simulink model "GPESTN1_GPEDBS"  (Simulink 6.1)
settings: Solver=ode45  StartTime=0.0  StopTime=1000.0  MaxStep=0.01  MinStep=0.005  RelTol=1e-3
values from neighbouring files (symbols this model uses):
  A_gpe = 2    [data_GPE.m]    (also in data_GPI.m)
  A_stn = 5    [data_GPI.m]    (also in data_STN.m)
  B_gpe = .08    (= 0.08)    [data_GPE.m]    (also in data_GPI.m)
  B_stn = 1    [data_GPI.m]    (also in data_STN.m)
  c_gpe = 1    [data_GPE.m]
  c_stn = 1    [data_STN.m]
  cag0 = i_v_16(177:192)    [launch_sysGPESTN1.m]    (also in launch_sysGPESTN1_GPEDBS.m)
  cas0 = i_v_16(65:80)    [launch_sysGPESTN1.m]    (also in launch_sysGPESTN1_GPEDBS.m)
  egpegpe = -80    [data_synapses.m]
  egpestn = -100    [data_synapses.m]
  ek_gpe = -80.0    (= -80)    [data_GPE.m]
  ek_stn = -80.0    (= -80)    [data_STN.m]
  el_gpe = -55.0    (= -55)    [data_GPE.m]
  el_stn = -60.0    (= -60)    [data_STN.m]
  epsil_gpe = 1*10^-4    (= 0.0001)    [data_GPE.m]
  epsil_stn = 3.75*10^-5    (= 3.75e-05)    [data_STN.m]
  estngpe = 0    [data_synapses.m]
  gahp_gpe = 30.0    (= 30)    [data_GPE.m]
  gahp_stn = 9.0    (= 9)    [data_STN.m]
  gca_gpe = 0.1    [data_GPE.m]
  gca_stn = 0.5    [data_STN.m]
  ggpegpe = .3    (= 0.3)    [data_synapses.m]    (also in launch_sysGPESTN1.m; launch_sysGPESTN1_GPEDBS.m = 0)
  ggpestn = .90    (= 0.9)    [data_synapses.m]
  gk_gpe = 30.0    (= 30)    [data_GPE.m]
  gk_stn = 45.0    (= 45)    [data_STN.m]
  gl_gpe = .1    (= 0.1)    [data_GPE.m]
  gl_stn = 2.25    [data_STN.m]
  gna_gpe = 120    [data_GPE.m]
  gna_stn = 37.5    [data_STN.m]
  gstngpe = .3    (= 0.3)    [data_synapses.m]
  gt_gpe = .5    (= 0.5)    [data_GPE.m]
  gt_stn = 0.5    [data_STN.m]
  hg0 = i_v_16(129:144)    [launch_sysGPESTN1.m]    (also in launch_sysGPESTN1_GPEDBS.m)
  hs0 = i_v_16(17:32)    [launch_sysGPESTN1.m]    (also in launch_sysGPESTN1_GPEDBS.m)
  k1_gpe = 30.0    (= 30)    [data_GPE.m]
  k1_stn = 15.0    (= 15)    [data_STN.m]
  kca_gpe = 15    [data_GPE.m]
  kca_stn = 22.5    [data_STN.m]
  ng0 = i_v_16(145:160)    [launch_sysGPESTN1.m]    (also in launch_sysGPESTN1_GPEDBS.m)
  ns0 = i_v_16(33:48)    [launch_sysGPESTN1.m]    (also in launch_sysGPESTN1_GPEDBS.m)
  phih_gpe = 0.05    [data_GPE.m]
  phih_stn = 0.75    [data_STN.m]
  phin_gpe = 0.1    [data_GPE.m]
  phin_stn = 0.75    [data_STN.m]
  phir_gpe = 1    [data_GPE.m]
  phir_stn = 0.5    [data_STN.m]
  rg0 = i_v_16(161:176)    [launch_sysGPESTN1.m]    (also in launch_sysGPESTN1_GPEDBS.m)
  rs0 = i_v_16(49:64)    [launch_sysGPESTN1.m]    (also in launch_sysGPESTN1_GPEDBS.m)
  sg0 = i_v_16(193:208)    [launch_sysGPESTN1.m]    (also in launch_sysGPESTN1_GPEDBS.m)
  sigmaa_gpe = 2    [data_GPE.m]
  sigmaa_stn = 7.8    [data_STN.m]
  sigmab_stn = -0.07    [data_STN.m]
  sigmagh_gpe = 2.0    (= 2)    [data_GPE.m]
  sigmagh_stn = 8.0    (= 8)    [data_STN.m]
  sigmah_gpe = -12    [data_GPE.m]
  sigmah_stn = -3.1    [data_STN.m]
  sigmam_gpe = 10.0    (= 10)    [data_GPE.m]
  sigmam_stn = 15.0    (= 15)    [data_STN.m]
  sigman_gpe = 14.0    (= 14)    [data_GPE.m]
  sigman_stn = 8.0    (= 8)    [data_STN.m]
  sigmar_gpe = -2.0    (= -2)    [data_GPE.m]
  sigmar_stn = -2.0    (= -2)    [data_STN.m]
  sigmas_gpe = 2    [data_GPE.m]
  sigmas_stn = 8.0    (= 8)    [data_STN.m]
  sigmatauh_gpe = -12    [data_GPE.m]
  sigmatauh_stn = -3.0    (= -3)    [data_STN.m]
  sigmataun_gpe = -12.0    (= -12)    [data_GPE.m]
  sigmataun_stn = -26.0    (= -26)    [data_STN.m]
  sigmataur_stn = -2.2    [data_STN.m]
  ss0 = i_v_16(81:96)    [launch_sysGPESTN1.m]    (also in launch_sysGPESTN1_GPEDBS.m)
  syn_stngpe_gain = .2    (= 0.2)    [data_STN.m]
  tauh0_gpe = .05    (= 0.05)    [data_GPE.m]
  tauh0_stn = 1.0    (= 1)    [data_STN.m]
  tauh1_gpe = .27    (= 0.27)    [data_GPE.m]
  tauh1_stn = 500.0    (= 500)    [data_STN.m]
  taun0_gpe = .05    (= 0.05)    [data_GPE.m]
  taun0_stn = 1.0    (= 1)    [data_STN.m]
  taun1_gpe = .27    (= 0.27)    [data_GPE.m]
  taun1_stn = 100.0    (= 100)    [data_STN.m]
  taur0_stn = 7.1    [data_STN.m]
  taur1_stn = 17.5    [data_STN.m]
  taur_gpe = 30.0    (= 30)    [data_GPE.m]
  theta_gpe = 20    [data_GPE.m]    (also in data_GPI.m)
  theta_stn = 30    [data_GPI.m]    (also in data_STN.m)
  thetaa_gpe = -57.0    (= -57)    [data_GPE.m]
  thetaa_stn = -63.0    (= -63)    [data_STN.m]
  thetab_stn = 0.25    [data_STN.m]
  thetagh_gpe = -57.0    (= -57)    [data_GPE.m]
  thetagh_stn = -39.0    (= -39)    [data_STN.m]
  thetah_gpe = -58.0    (= -58)    [data_GPE.m]
  thetah_stn = -39.0    (= -39)    [data_STN.m]
  thetam_gpe = -37.0    (= -37)    [data_GPE.m]
  thetam_stn = -30.0    (= -30)    [data_STN.m]
  thetan_gpe = -50.0    (= -50)    [data_GPE.m]
  thetan_stn = -32.0    (= -32)    [data_STN.m]
  thetar_gpe = -70.0    (= -70)    [data_GPE.m]
  thetar_stn = -67.0    (= -67)    [data_STN.m]
  thetas_gpe = -35.0    (= -35)    [data_GPE.m]
  thetas_stn = -39.0    (= -39)    [data_STN.m]
  thetatauh_gpe = -40.0    (= -40)    [data_GPE.m]
  thetatauh_stn = -57.0    (= -57)    [data_STN.m]
  thetataun_gpe = -40.0    (= -40)    [data_GPE.m]
  thetataun_stn = -80.0    (= -80)    [data_STN.m]
  thetataur_stn = 68.0    (= 68)    [data_STN.m]
  vg0 = i_v_16(113:128)    [launch_sysGPESTN1.m]    (also in launch_sysGPESTN1_GPEDBS.m)
  vs0 = i_v_16(1:16)    [launch_sysGPESTN1.m]    (also in launch_sysGPESTN1_GPEDBS.m)
undefined symbols (not defined in the file or in its folder): cag01, cas01, hg01, hs01, ng01, ns01, rg01, rs01, sg01, ss01, vg01, vs01
(part 1 of 9)
settings Model: LastModifiedBy=marco  ExtModeAutoUpdateStatusClock=off
settings DataIOCC: SignalLoggingName=sigsOut
settings OptimizationCC: BooleanDataType=off  InlineInvariantSignals=off
settings HardwareCC: TargetUnknown=on

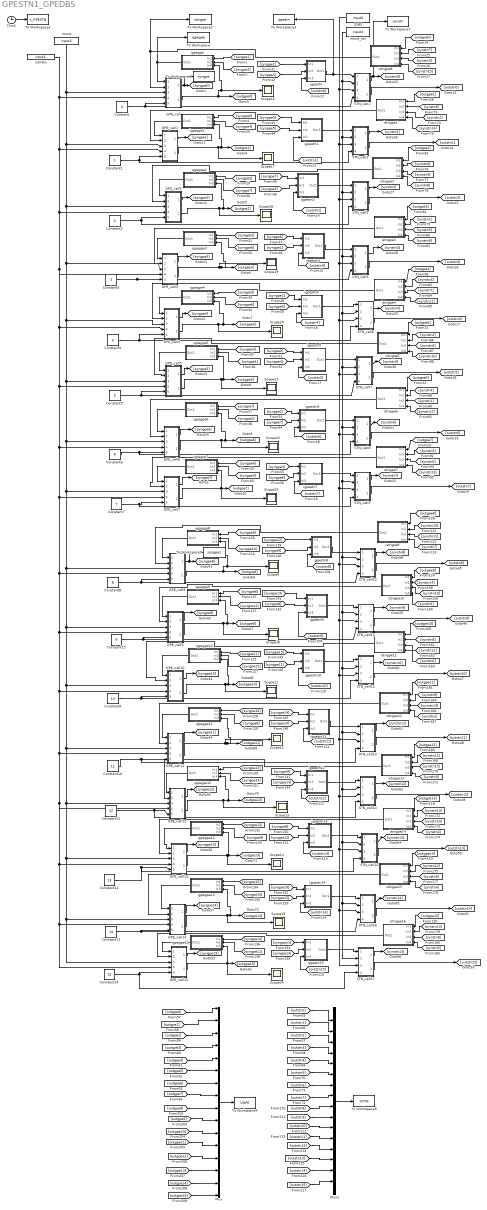
== system GPESTN1_GPEDBS ==
  Clock : Clock
      settings: Decimation=10
  Constant : Constant  Value=0
  Constant1 : Constant
  Constant10 : Constant  Value=11
  Constant11 : Constant  Value=12
  Constant12 : Constant  Value=13
  Constant13 : Constant  Value=14
  Constant14 : Constant  Value=15
  Constant15 : Constant  Value=9
  Constant2 : Constant  Value=2
  Constant3 : Constant  Value=3
  Constant4 : Constant  Value=4
  Constant5 : Constant  Value=5
  Constant6 : Constant  Value=6
  Constant7 : Constant  Value=7
  Constant8 : Constant  Value=8
  Constant9 : Constant  Value=10
  GPE_cell : Subsystem
  GPE_cell1 : Subsystem
  GPE_cell10 : Subsystem
  GPE_cell11 : Subsystem
  GPE_cell12 : Subsystem
  GPE_cell13 : Subsystem
  GPE_cell14 : Subsystem
  GPE_cell15 : Subsystem
  GPE_cell2 : Subsystem
  GPE_cell3 : Subsystem
  GPE_cell4 : Subsystem
  GPE_cell5 : Subsystem
  GPE_cell6 : Subsystem
  GPE_cell7 : Subsystem
  GPE_cell8 : Subsystem
  GPE_cell9 : Subsystem
  IDBS : FromWorkspace  Orientation=left  VariableName=input3  SampleTime=0.01
  Mux : Mux  Inputs=16
  Mux1 : Mux  Inputs=16
  STN_cell1 : Subsystem
  STN_cell10 : Subsystem
  STN_cell11 : Subsystem
  STN_cell12 : Subsystem
  STN_cell13 : Subsystem
  STN_cell14 : Subsystem
  STN_cell15 : Subsystem
  STN_cell16 : Subsystem
  STN_cell17 : Subsystem
  STN_cell2 : Subsystem
  STN_cell3 : Subsystem
  STN_cell5 : Subsystem
  STN_cell6 : Subsystem
  STN_cell7 : Subsystem
  STN_cell8 : Subsystem
  STN_cell9 : Subsystem
  Scope{9..24} (16 alike) : Scope
      Scope10 settings: YMin=-125  YMax=75  SaveName=ScopeData9
      Scope11 settings: YMin=-80  YMax=60  SaveName=ScopeData10
      Scope12 settings: YMin=-250  YMax=100  SaveName=ScopeData11
      Scope13 settings: YMin=-100  YMax=60  SaveName=ScopeData12
      Scope14 settings: YMin=-80  YMax=60  SaveName=ScopeData13
      Scope15 settings: YMin=-250  YMax=100  SaveName=ScopeData14
      Scope16 settings: YMin=-80  YMax=60
      Scope17 settings: YMin=-80  YMax=60  SaveName=ScopeData16
      Scope18 settings: YMin=-80  YMax=60  SaveName=ScopeData17
      Scope19 settings: YMin=-80  YMax=60  SaveName=ScopeData18
      Scope20 settings: SaveName=ScopeData19
      Scope21 settings: YMin=-80  YMax=60  SaveName=ScopeData20
      Scope22 settings: YMin=-80  YMax=60  SaveName=ScopeData21
      Scope23 settings: YMin=-80  YMax=60  SaveName=ScopeData22
      Scope24 settings: YMin=-80  YMax=60  SaveName=ScopeData15
      Scope9 settings: YMin=-90  YMax=60  SaveName=ScopeData23
  To Workspace : ToWorkspace  VariableName=igpegpe  SampleTime=-1  SaveFormat=Array
  To Workspace1 : ToWorkspace  VariableName=t_GPESTN  SampleTime=-1  SaveFormat=Array
  To Workspace2 : ToWorkspace  VariableName=istngpe  SampleTime=-1  SaveFormat=Array
  To Workspace3 : ToWorkspace  VariableName=igpestn  SampleTime=-1  SaveFormat=Array
  To Workspace4 : ToWorkspace  VariableName=VGPE  SampleTime=-1  SaveFormat=Array
  To Workspace5 : ToWorkspace  VariableName=VSTN  SampleTime=-1  SaveFormat=Array
  To Workspace6 : ToWorkspace  VariableName=syngpe  SampleTime=-1  SaveFormat=Array
  To Workspace7 : ToWorkspace  VariableName=synstn  SampleTime=-1  SaveFormat=Array
  To Workspace9 : ToWorkspace  VariableName=syngpe1  SampleTime=-1  SaveFormat=Array
  igpegpe : Subsystem  Orientation=left
  igpegpe1 : Subsystem  Orientation=left
  igpegpe10 : Subsystem  Orientation=left
  igpegpe11 : Subsystem  Orientation=left
  igpegpe12 : Subsystem  Orientation=left
  igpegpe13 : Subsystem  Orientation=left
  igpegpe14 : Subsystem  Orientation=left
  igpegpe15 : Subsystem  Orientation=left
  igpegpe2 : Subsystem  Orientation=left
  igpegpe3 : Subsystem  Orientation=left
  igpegpe4 : Subsystem  Orientation=left
  igpegpe5 : Subsystem  Orientation=left
  igpegpe6 : Subsystem  Orientation=left
  igpegpe7 : Subsystem  Orientation=left
  igpegpe8 : Subsystem  Orientation=left
  igpegpe9 : Subsystem  Orientation=left
  igpestn : Subsystem
  igpestn1 : Subsystem
  igpestn10 : Subsystem
  igpestn11 : Subsystem
  igpestn12 : Subsystem
  igpestn13 : Subsystem
  igpestn14 : Subsystem
  igpestn15 : Subsystem
  igpestn2 : Subsystem
  igpestn3 : Subsystem
  igpestn4 : Subsystem
  igpestn5 : Subsystem
  igpestn6 : Subsystem
  igpestn7 : Subsystem
  igpestn8 : Subsystem
  igpestn9 : Subsystem
  imore : FromWorkspace  Orientation=down  VariableName=input2  SampleTime=1
  imore_stn : FromWorkspace  Orientation=left  VariableName=input4  SampleTime=1
  istngpe1 : Subsystem  Orientation=left
  istngpe10 : Subsystem  Orientation=left
  istngpe11 : Subsystem  Orientation=left
  istngpe12 : Subsystem  Orientation=left
  istngpe13 : Subsystem  Orientation=left
  istngpe14 : Subsystem  Orientation=left
  istngpe15 : Subsystem  Orientation=left
  istngpe16 : Subsystem  Orientation=left
  istngpe2 : Subsystem  Orientation=left
  istngpe3 : Subsystem  Orientation=left
  istngpe4 : Subsystem  Orientation=left
  istngpe5 : Subsystem  Orientation=left
  istngpe6 : Subsystem  Orientation=left
  istngpe7 : Subsystem  Orientation=left
  istngpe8 : Subsystem  Orientation=left
  istngpe9 : Subsystem  Orientation=left
  istriato : FromWorkspace  VariableName=input1  SampleTime=1
  wires:
  Clock/1 -> To Workspace1/1
  istriato/1 -> GPE_cell14/4(In4), GPE_cell15/4(In4), GPE_cell13/4(In4), GPE_cell12/4(In4), GPE_cell11/4(In4), GPE_cell10/4(In4), GPE_cell9/4(In4), GPE_cell8/4(In4), GPE_cell7/4(In4), GPE_cell6/4(In4), GPE_cell5/4(In4), GPE_cell4/4(In4), GPE_cell3/4(In4), GPE_cell2/4(In4), GPE_cell1/4(In4), GPE_cell/4(In4)
  imore/1 -> GPE_cell/3(In3), GPE_cell14/3(In3), GPE_cell15/3(In3), GPE_cell13/3(In3), GPE_cell12/3(In3), GPE_cell11/3(In3), GPE_cell10/3(In3), GPE_cell9/3(In3), GPE_cell8/3(In3), GPE_cell7/3(In3), GPE_cell6/3(In3), GPE_cell5/3(In3), GPE_cell4/3(In3), GPE_cell3/3(In3), GPE_cell2/3(In3), GPE_cell1/3(In3)
  GPE_cell7/1(Out1) -> [syngpe7]
  igpegpe/1(Out1) -> To Workspace/1, GPE_cell/1(In1)
  GPE_cell/1(Out1) -> [syngpe0], To Workspace6/1
  igpegpe2/1(Out1) -> GPE_cell2/1(In1)
  igpegpe3/1(Out1) -> GPE_cell3/1(In1)
  igpegpe4/1(Out1) -> GPE_cell4/1(In1)
  igpegpe5/1(Out1) -> GPE_cell5/1(In1)
  igpegpe6/1(Out1) -> GPE_cell6/1(In1)
  igpegpe7/1(Out1) -> GPE_cell7/1(In1)
  imore_stn/1 -> STN_cell16/2(In2), STN_cell17/2(In2), STN_cell15/2(In2), STN_cell14/2(In2), STN_cell13/2(In2), STN_cell12/2(In2), STN_cell11/2(In2), STN_cell10/2(In2), STN_cell9/2(In2), STN_cell8/2(In2), STN_cell7/2(In2), STN_cell6/2(In2), STN_cell5/2(In2), STN_cell3/2(In2), STN_cell2/2(In2), STN_cell1/2(In2)
  IDBS/1 -> STN_cell16/3(In3), STN_cell17/3(In3), STN_cell15/3(In3), STN_cell14/3(In3), STN_cell13/3(In3), STN_cell12/3(In3), STN_cell11/3(In3), STN_cell10/3(In3), STN_cell9/3(In3), STN_cell8/3(In3), STN_cell7/3(In3), STN_cell6/3(In3), STN_cell5/3(In3), STN_cell3/3(In3), STN_cell2/3(In3), STN_cell1/3(In3)
  GPE_cell/2(Out2) -> [outgpe0], Scope16/1, igpegpe/3(In3)
  GPE_cell1/2(Out2) -> Scope17/1, [outgpe1], igpegpe1/3(In3)
  GPE_cell2/2(Out2) -> Scope18/1, [outgpe2], igpegpe2/3(In3)
  GPE_cell3/2(Out2) -> Scope19/1, [outgpe3], igpegpe3/3(In3)
  GPE_cell4/2(Out2) -> Scope20/1, [outgpe4], igpegpe4/3(In3)
  GPE_cell5/2(Out2) -> Scope21/1, [outgpe5], igpegpe5/3(In3)
  GPE_cell6/2(Out2) -> Scope22/1, [outgpe6], igpegpe6/3(In3)
  GPE_cell7/2(Out2) -> [outgpe7], Scope23/1, igpegpe7/3(In3)
  istngpe3/1(Out1) -> GPE_cell3/2(In2)
  igpestn/1(Out1) -> To Workspace3/1, STN_cell1/1(In1)
  [outstn0] -> igpestn/3(In3)
  [outstn1] -> igpestn1/3(In3)
  igpestn1/1(Out1) -> STN_cell2/1(In1)
  igpestn2/1(Out1) -> STN_cell3/1(In1)
  [outstn2] -> igpestn2/3(In3)
  igpestn3/1(Out1) -> STN_cell5/1(In1)
  [outstn3] -> igpestn3/3(In3)
  igpestn4/1(Out1) -> STN_cell6/1(In1)
  [outstn4] -> igpestn4/3(In3)
  igpestn5/1(Out1) -> STN_cell7/1(In1)
  [outstn5] -> igpestn5/3(In3)
  igpestn6/1(Out1) -> STN_cell8/1(In1)
  [outstn6] -> igpestn6/3(In3)
  igpestn7/1(Out1) -> STN_cell9/1(In1)
  [outstn7] -> igpestn7/3(In3)
  GPE_cell1/1(Out1) -> [syngpe1]
  GPE_cell2/1(Out1) -> [syngpe2]
  GPE_cell3/1(Out1) -> [syngpe3]
  GPE_cell4/1(Out1) -> [syngpe4]
  GPE_cell5/1(Out1) -> [syngpe5]
  GPE_cell6/1(Out1) -> [syngpe6]
  [syngpe1] -> igpegpe/1(In1)
  [syngpe2] -> igpegpe/2(In2)
  [syngpe0] -> igpegpe1/1(In1)
  [syngpe4] -> igpegpe1/2(In2)
  [syngpe3] -> igpegpe2/1(In1)
  [syngpe7] -> igpegpe2/2(In2)
  [syngpe2] -> igpegpe3/1(In1)
  [syngpe0] -> igpegpe3/2(In2)
  [syngpe5] -> igpegpe4/1(In1)
  [syngpe6] -> igpegpe4/2(In2)
  [syngpe4] -> igpegpe5/1(In1)
  [syngpe1] -> igpegpe5/2(In2)
  [syngpe7] -> igpegpe6/1(In1)
  [syngpe2] -> igpegpe6/2(In2)
  [syngpe6] -> igpegpe7/1(In1)
  [syngpe3] -> igpegpe7/2(In2)
  [syngpe1] -> igpestn/1(In1)
  [syngpe4] -> igpestn/2(In2)
  [syngpe0] -> igpestn1/1(In1)
  [syngpe5] -> igpestn1/2(In2)
  [syngpe7] -> igpestn2/1(In1)
  [syngpe3] -> igpestn2/2(In2)
  [syngpe6] -> igpestn3/1(In1)
  [syngpe2] -> igpestn3/2(In2)
  [syngpe1] -> igpestn4/1(In1)
  [syngpe5] -> igpestn4/2(In2)
  [syngpe0] -> igpestn5/1(In1)
  [syngpe4] -> igpestn5/2(In2)
  [syngpe2] -> igpestn6/1(In1)
  [syngpe7] -> igpestn6/2(In2)
  [syngpe3] -> igpestn7/1(In1)
  [syngpe6] -> igpestn7/2(In2)
  [outgpe0] -> Mux/1
  [outgpe1] -> Mux/2
  [outgpe2] -> Mux/3
  [outgpe3] -> Mux/4
  [outgpe4] -> Mux/5
  [outgpe5] -> Mux/6
  [outgpe6] -> Mux/7
  [outgpe7] -> Mux/8
  [outstn0] -> Mux1/1
  [outstn1] -> Mux1/2
  [outstn2] -> Mux1/3
  [outstn3] -> Mux1/4
  [outstn4] -> Mux1/5
  [outstn5] -> Mux1/6
  [outstn6] -> Mux1/7
  [outstn7] -> Mux1/8
  Mux/1 -> To Workspace4/1
  Mux1/1 -> To Workspace5/1
  STN_cell1/2(Out2) -> [outstn0]
  STN_cell2/2(Out2) -> [outstn1]
  STN_cell8/2(Out2) -> [outstn6]
  STN_cell7/2(Out2) -> [outstn5]
  STN_cell5/2(Out2) -> [outstn3]
  STN_cell3/2(Out2) -> [outstn2]
  [outgpe0] -> istngpe8/1(In1)
  [outgpe1] -> istngpe1/1(In1)
  STN_cell1/1(Out1) -> [synstn0], To Workspace7/1
  STN_cell9/1(Out1) -> [synstn7]
  STN_cell8/1(Out1) -> [synstn6]
  STN_cell7/1(Out1) -> [synstn5]
  STN_cell6/1(Out1) -> [synstn4]
  STN_cell5/1(Out1) -> [synstn3]
  STN_cell2/1(Out1) -> [synstn1]
  STN_cell3/1(Out1) -> [synstn2]
  [outgpe4] -> istngpe4/1(In1)
  [outgpe5] -> istngpe5/1(In1)
  [outgpe6] -> istngpe6/1(In1)
  [outgpe7] -> istngpe7/1(In1)
  [synstn7] -> istngpe8/2(In2)
  [synstn3] -> istngpe8/3(In3)
  [synstn15] -> istngpe8/4(In4)
  [synstn6] -> istngpe1/2(In2)
  [synstn14] -> istngpe1/4(In4)
  [synstn3] -> istngpe4/2(In2)
  [synstn7] -> istngpe4/3(In3)
  [synstn11] -> istngpe4/4(In4)
  [synstn4] -> istngpe6/2(In2)
  [synstn1] -> istngpe6/3(In3)
  [synstn12] -> istngpe6/4(In4)
  [synstn5] -> istngpe7/2(In2)
  [synstn0] -> istngpe7/3(In3)
  [synstn13] -> istngpe7/4(In4)
  STN_cell6/2(Out2) -> [outstn4]
  STN_cell9/2(Out2) -> [outstn7]
  istngpe4/1(Out1) -> GPE_cell4/2(In2)
  istngpe5/1(Out1) -> GPE_cell5/2(In2)
  istngpe6/1(Out1) -> GPE_cell6/2(In2)
  istngpe7/1(Out1) -> GPE_cell7/2(In2)
  istngpe2/1(Out1) -> GPE_cell2/2(In2)
  istngpe8/1(Out1) -> To Workspace2/1, GPE_cell/2(In2)
  [synstn2] -> istngpe1/3(In3)
  [outgpe2] -> istngpe2/1(In1)
  [synstn0] -> istngpe2/2(In2)
  [synstn4] -> istngpe2/3(In3)
  [synstn8] -> istngpe2/4(In4)
  [outgpe3] -> istngpe3/1(In1)
  [synstn1] -> istngpe3/2(In2)
  [synstn5] -> istngpe3/3(In3)
  [synstn9] -> istngpe3/4(In4)
  [synstn2] -> istngpe5/2(In2)
  [synstn6] -> istngpe5/3(In3)
  [synstn10] -> istngpe5/4(In4)
  GPE_cell15/1(Out1) -> [syngpe15]
  igpegpe8/1(Out1) -> GPE_cell8/1(In1)
  GPE_cell8/1(Out1) -> [syngpe8], To Workspace9/1
  igpegpe10/1(Out1) -> GPE_cell10/1(In1)
  igpegpe9/1(Out1) -> GPE_cell9/1(In1)
  igpegpe11/1(Out1) -> GPE_cell11/1(In1)
  igpegpe12/1(Out1) -> GPE_cell12/1(In1)
  igpegpe13/1(Out1) -> GPE_cell13/1(In1)
  igpegpe14/1(Out1) -> GPE_cell14/1(In1)
  igpegpe15/1(Out1) -> GPE_cell15/1(In1)
  GPE_cell8/2(Out2) -> [outgpe8], Scope9/1, igpegpe8/3(In3)
  GPE_cell9/2(Out2) -> Scope10/1, [outgpe9], igpegpe9/3(In3)
  GPE_cell10/2(Out2) -> Scope11/1, [outgpe10], igpegpe10/3(In3)
  GPE_cell11/2(Out2) -> Scope12/1, [outgpe11], igpegpe11/3(In3)
  GPE_cell12/2(Out2) -> Scope13/1, [outgpe12], igpegpe12/3(In3)
  GPE_cell13/2(Out2) -> Scope14/1, [outgpe13], igpegpe13/3(In3)
  GPE_cell14/2(Out2) -> Scope15/1, [outgpe14], igpegpe14/3(In3)
  GPE_cell15/2(Out2) -> [outgpe15], Scope24/1, igpegpe15/3(In3)
  istngpe12/1(Out1) -> GPE_cell11/2(In2)
  igpestn8/1(Out1) -> STN_cell10/1(In1)
  [outstn8] -> igpestn8/3(In3)
  [outstn9] -> igpestn9/3(In3)
  igpestn9/1(Out1) -> STN_cell11/1(In1)
  igpestn10/1(Out1) -> STN_cell12/1(In1)
  [outstn10] -> igpestn10/3(In3)
  igpestn11/1(Out1) -> STN_cell13/1(In1)
  [outstn11] -> igpestn11/3(In3)
  igpestn12/1(Out1) -> STN_cell14/1(In1)
  [outstn12] -> igpestn12/3(In3)
  igpestn13/1(Out1) -> STN_cell15/1(In1)
  [outstn13] -> igpestn13/3(In3)
  igpestn14/1(Out1) -> STN_cell16/1(In1)
  [outstn14] -> igpestn14/3(In3)
  igpestn15/1(Out1) -> STN_cell17/1(In1)
  [outstn15] -> igpestn15/3(In3)
  GPE_cell9/1(Out1) -> [syngpe9]
  GPE_cell10/1(Out1) -> [syngpe10]
  GPE_cell11/1(Out1) -> [syngpe11]
  GPE_cell12/1(Out1) -> [syngpe12]
  GPE_cell13/1(Out1) -> [syngpe13]
  GPE_cell14/1(Out1) -> [syngpe14]
  [syngpe9] -> igpegpe8/1(In1)
  [syngpe10] -> igpegpe8/2(In2)
  [syngpe8] -> igpegpe9/1(In1)
  [syngpe12] -> igpegpe9/2(In2)
  [syngpe11] -> igpegpe10/1(In1)
  [syngpe15] -> igpegpe10/2(In2)
  [syngpe10] -> igpegpe11/1(In1)
  [syngpe8] -> igpegpe11/2(In2)
  [syngpe13] -> igpegpe12/1(In1)
  [syngpe14] -> igpegpe12/2(In2)
  [syngpe12] -> igpegpe13/1(In1)
  [syngpe9] -> igpegpe13/2(In2)
  [syngpe15] -> igpegpe14/1(In1)
  [syngpe10] -> igpegpe14/2(In2)
  [syngpe14] -> igpegpe15/1(In1)
  [syngpe11] -> igpegpe15/2(In2)
  [syngpe12] -> igpestn8/1(In1)
  [syngpe9] -> igpestn8/2(In2)
  [syngpe13] -> igpestn9/1(In1)
  [syngpe8] -> igpestn9/2(In2)
  [syngpe15] -> igpestn10/1(In1)
  [syngpe11] -> igpestn10/2(In2)
  [syngpe14] -> igpestn11/1(In1)
  [syngpe10] -> igpestn11/2(In2)
  [syngpe9] -> igpestn12/1(In1)
  [syngpe13] -> igpestn12/2(In2)
  [syngpe8] -> igpestn13/1(In1)
  [syngpe12] -> igpestn13/2(In2)
  [syngpe10] -> igpestn14/1(In1)
  [syngpe15] -> igpestn14/2(In2)
  [syngpe11] -> igpestn15/1(In1)
  [syngpe14] -> igpestn15/2(In2)
  STN_cell10/2(Out2) -> [outstn8]
  STN_cell11/2(Out2) -> [outstn9]
  STN_cell16/2(Out2) -> [outstn14]
  STN_cell15/2(Out2) -> [outstn13]
  STN_cell13/2(Out2) -> [outstn11]
  STN_cell12/2(Out2) -> [outstn10]
  [outgpe9] -> istngpe10/1(In1)
  STN_cell10/1(Out1) -> [synstn8]
  STN_cell17/1(Out1) -> [synstn15]
  STN_cell16/1(Out1) -> [synstn14]
  STN_cell15/1(Out1) -> [synstn13]
  STN_cell14/1(Out1) -> [synstn12]
  STN_cell13/1(Out1) -> [synstn11]
  STN_cell11/1(Out1) -> [synstn9]
  STN_cell12/1(Out1) -> [synstn10]
  [outgpe12] -> istngpe13/1(In1)
  [outgpe13] -> istngpe14/1(In1)
  [outgpe14] -> istngpe15/1(In1)
  [outgpe15] -> istngpe16/1(In1)
  [synstn15] -> istngpe9/2(In2)
  [synstn11] -> istngpe9/3(In3)
  [synstn7] -> istngpe9/4(In4)
  [synstn14] -> istngpe10/2(In2)
  [synstn6] -> istngpe10/4(In4)
  [synstn11] -> istngpe13/2(In2)
  [synstn15] -> istngpe13/3(In3)
  [synstn3] -> istngpe13/4(In4)
  [synstn12] -> istngpe15/2(In2)
  [synstn9] -> istngpe15/3(In3)
  [synstn4] -> istngpe15/4(In4)
  [synstn13] -> istngpe16/2(In2)
  [synstn8] -> istngpe16/3(In3)
  [synstn5] -> istngpe16/4(In4)
  STN_cell14/2(Out2) -> [outstn12]
  STN_cell17/2(Out2) -> [outstn15]
  istngpe13/1(Out1) -> GPE_cell12/2(In2)
  istngpe15/1(Out1) -> GPE_cell14/2(In2)
  istngpe16/1(Out1) -> GPE_cell15/2(In2)
  istngpe11/1(Out1) -> GPE_cell10/2(In2)
  istngpe10/1(Out1) -> GPE_cell9/2(In2)
  istngpe9/1(Out1) -> GPE_cell8/2(In2)
  [synstn10] -> istngpe10/3(In3)
  [outgpe10] -> istngpe11/1(In1)
  [synstn8] -> istngpe11/2(In2)
  [synstn12] -> istngpe11/3(In3)
  [synstn0] -> istngpe11/4(In4)
  [outgpe11] -> istngpe12/1(In1)
  [synstn9] -> istngpe12/2(In2)
  [synstn13] -> istngpe12/3(In3)
  [synstn1] -> istngpe12/4(In4)
  [synstn10] -> istngpe14/2(In2)
  [synstn14] -> istngpe14/3(In3)
  [synstn2] -> istngpe14/4(In4)
  [outgpe8] -> Mux/9
  [outgpe9] -> Mux/10
  [outgpe10] -> Mux/11
  [outgpe11] -> Mux/12
  [outgpe12] -> Mux/13
  [outgpe13] -> Mux/14
  [outgpe14] -> Mux/15
  [outgpe15] -> Mux/16
  [outstn8] -> Mux1/9
  [outstn9] -> Mux1/10
  [outstn10] -> Mux1/11
  [outstn11] -> Mux1/12
  [outstn12] -> Mux1/13
  [outstn13] -> Mux1/14
  [outstn14] -> Mux1/15
  [outstn15] -> Mux1/16
  [outgpe8] -> istngpe9/1(In1)
  igpegpe1/1(Out1) -> GPE_cell1/1(In1)
  istngpe1/1(Out1) -> GPE_cell1/2(In2)
  Constant/1 -> GPE_cell/5(In5), STN_cell1/4(In4)
  Constant1/1 -> GPE_cell1/5(In5), STN_cell2/4(In4)
  Constant2/1 -> GPE_cell2/5(In5), STN_cell3/4(In4)
  Constant3/1 -> GPE_cell3/5(In5), STN_cell5/4(In4)
  Constant4/1 -> GPE_cell4/5(In5), STN_cell6/4(In4)
  Constant5/1 -> GPE_cell5/5(In5), STN_cell7/4(In4)
  Constant6/1 -> GPE_cell6/5(In5), STN_cell8/4(In4)
  Constant7/1 -> GPE_cell7/5(In5), STN_cell9/4(In4)
  Constant8/1 -> GPE_cell8/5(In5), STN_cell10/4(In4)
  Constant15/1 -> GPE_cell9/5(In5), STN_cell11/4(In4)
  Constant9/1 -> GPE_cell10/5(In5), STN_cell12/4(In4)
  Constant10/1 -> GPE_cell11/5(In5), STN_cell13/4(In4)
  Constant11/1 -> GPE_cell12/5(In5), STN_cell14/4(In4)
  Constant12/1 -> GPE_cell13/5(In5), STN_cell15/4(In4)
  Constant13/1 -> GPE_cell14/5(In5), STN_cell16/4(In4)
  Constant14/1 -> GPE_cell15/5(In5), STN_cell17/4(In4)
  istngpe14/1(Out1) -> GPE_cell13/2(In2)

== system GPESTN1_GPEDBS/GPE_cell ==
  In1 : Inport  Port=1  LatchInput=off
  In2 : Inport  Port=2  LatchInput=off
  In3 : Inport  Port=3  LatchInput=off
  In4 : Inport  Port=4  LatchInput=off
  In5 : Inport  Port=5  LatchInput=off
  Constant : Constant  Value=sg0
  Selector5 : Selector  IndexMode=Zero-based  ElementSrc=External  Elements=[1 3]
  gpe_cell : Subsystem
  synap_gpe : Subsystem
  Out1 : Outport
  Out2 : Outport  Port=2
  wires:
  gpe_cell/1(Out1) -> synap_gpe/1(In1), Out2/1
  In3/1 -> gpe_cell/3(In3)
  In4/1 -> gpe_cell/4(In4)
  synap_gpe/1(Out1) -> Out1/1
  In1/1 -> gpe_cell/1(In1)
  In2/1 -> gpe_cell/2(In2)
  Selector5/1 -> synap_gpe/2(In2)
  In5/1 -> gpe_cell/5(In5), Selector5/2
  Constant/1 -> Selector5/1

== system GPESTN1_GPEDBS/GPE_cell1 ==
  In1 : Inport  Port=1  LatchInput=off
  In2 : Inport  Port=2  LatchInput=off
  In3 : Inport  Port=3  LatchInput=off
  In4 : Inport  Port=4  LatchInput=off
  In5 : Inport  Port=5  LatchInput=off
  Constant : Constant  Value=sg0
  Selector5 : Selector  IndexMode=Zero-based  ElementSrc=External  Elements=[1 3]
  gpe_cell : Subsystem
  synap_gpe : Subsystem
  Out1 : Outport
  Out2 : Outport  Port=2
  wires:
  gpe_cell/1(Out1) -> synap_gpe/1(In1), Out2/1
  In3/1 -> gpe_cell/3(In3)
  In4/1 -> gpe_cell/4(In4)
  synap_gpe/1(Out1) -> Out1/1
  In1/1 -> gpe_cell/1(In1)
  In2/1 -> gpe_cell/2(In2)
  Selector5/1 -> synap_gpe/2(In2)
  In5/1 -> gpe_cell/5(In5), Selector5/2
  Constant/1 -> Selector5/1

== system GPESTN1_GPEDBS/GPE_cell10 ==
  In1 : Inport  Port=1  LatchInput=off
  In2 : Inport  Port=2  LatchInput=off
  In3 : Inport  Port=3  LatchInput=off
  In4 : Inport  Port=4  LatchInput=off
  In5 : Inport  Port=5  LatchInput=off
  Constant : Constant  Value=sg0
  Selector5 : Selector  IndexMode=Zero-based  ElementSrc=External  Elements=[1 3]
  gpe_cell : Subsystem
  synap_gpe : Subsystem
  Out1 : Outport
  Out2 : Outport  Port=2
  wires:
  gpe_cell/1(Out1) -> synap_gpe/1(In1), Out2/1
  In3/1 -> gpe_cell/3(In3)
  In4/1 -> gpe_cell/4(In4)
  synap_gpe/1(Out1) -> Out1/1
  In1/1 -> gpe_cell/1(In1)
  In2/1 -> gpe_cell/2(In2)
  Selector5/1 -> synap_gpe/2(In2)
  In5/1 -> gpe_cell/5(In5), Selector5/2
  Constant/1 -> Selector5/1

== system GPESTN1_GPEDBS/GPE_cell11 ==
  In1 : Inport  Port=1  LatchInput=off
  In2 : Inport  Port=2  LatchInput=off
  In3 : Inport  Port=3  LatchInput=off
  In4 : Inport  Port=4  LatchInput=off
  In5 : Inport  Port=5  LatchInput=off
  Constant : Constant  Value=sg0
  Selector5 : Selector  IndexMode=Zero-based  ElementSrc=External  Elements=[1 3]
  gpe_cell : Subsystem
  synap_gpe : Subsystem
  Out1 : Outport
  Out2 : Outport  Port=2
  wires:
  gpe_cell/1(Out1) -> synap_gpe/1(In1), Out2/1
  In3/1 -> gpe_cell/3(In3)
  In4/1 -> gpe_cell/4(In4)
  synap_gpe/1(Out1) -> Out1/1
  In1/1 -> gpe_cell/1(In1)
  In2/1 -> gpe_cell/2(In2)
  Selector5/1 -> synap_gpe/2(In2)
  In5/1 -> gpe_cell/5(In5), Selector5/2
  Constant/1 -> Selector5/1

== system GPESTN1_GPEDBS/GPE_cell12 ==
  In1 : Inport  Port=1  LatchInput=off
  In2 : Inport  Port=2  LatchInput=off
  In3 : Inport  Port=3  LatchInput=off
  In4 : Inport  Port=4  LatchInput=off
  In5 : Inport  Port=5  LatchInput=off
  Constant : Constant  Value=sg0
  Selector5 : Selector  IndexMode=Zero-based  ElementSrc=External  Elements=[1 3]
  gpe_cell : Subsystem
  synap_gpe : Subsystem
  Out1 : Outport
  Out2 : Outport  Port=2
  wires:
  gpe_cell/1(Out1) -> synap_gpe/1(In1), Out2/1
  In3/1 -> gpe_cell/3(In3)
  In4/1 -> gpe_cell/4(In4)
  synap_gpe/1(Out1) -> Out1/1
  In1/1 -> gpe_cell/1(In1)
  In2/1 -> gpe_cell/2(In2)
  Selector5/1 -> synap_gpe/2(In2)
  In5/1 -> gpe_cell/5(In5), Selector5/2
  Constant/1 -> Selector5/1

== system GPESTN1_GPEDBS/GPE_cell13 ==
  In1 : Inport  Port=1  LatchInput=off
  In2 : Inport  Port=2  LatchInput=off
  In3 : Inport  Port=3  LatchInput=off
  In4 : Inport  Port=4  LatchInput=off
  In5 : Inport  Port=5  LatchInput=off
  Constant : Constant  Value=sg0
  Selector5 : Selector  IndexMode=Zero-based  ElementSrc=External  Elements=[1 3]
  gpe_cell : Subsystem
  synap_gpe : Subsystem
  Out1 : Outport
  Out2 : Outport  Port=2
  wires:
  gpe_cell/1(Out1) -> synap_gpe/1(In1), Out2/1
  In3/1 -> gpe_cell/3(In3)
  In4/1 -> gpe_cell/4(In4)
  synap_gpe/1(Out1) -> Out1/1
  In1/1 -> gpe_cell/1(In1)
  In2/1 -> gpe_cell/2(In2)
  Selector5/1 -> synap_gpe/2(In2)
  In5/1 -> gpe_cell/5(In5), Selector5/2
  Constant/1 -> Selector5/1

== system GPESTN1_GPEDBS/GPE_cell14 ==
  In1 : Inport  Port=1  LatchInput=off
  In2 : Inport  Port=2  LatchInput=off
  In3 : Inport  Port=3  LatchInput=off
  In4 : Inport  Port=4  LatchInput=off
  In5 : Inport  Port=5  LatchInput=off
  Constant : Constant  Value=sg0
  Selector5 : Selector  IndexMode=Zero-based  ElementSrc=External  Elements=[1 3]
  gpe_cell : Subsystem
  synap_gpe : Subsystem
  Out1 : Outport
  Out2 : Outport  Port=2
  wires:
  gpe_cell/1(Out1) -> synap_gpe/1(In1), Out2/1
  In3/1 -> gpe_cell/3(In3)
  In4/1 -> gpe_cell/4(In4)
  synap_gpe/1(Out1) -> Out1/1
  In1/1 -> gpe_cell/1(In1)
  In2/1 -> gpe_cell/2(In2)
  Selector5/1 -> synap_gpe/2(In2)
  In5/1 -> gpe_cell/5(In5), Selector5/2
  Constant/1 -> Selector5/1

== system GPESTN1_GPEDBS/GPE_cell15 ==
  In1 : Inport  Port=1  LatchInput=off
  In2 : Inport  Port=2  LatchInput=off
  In3 : Inport  Port=3  LatchInput=off
  In4 : Inport  Port=4  LatchInput=off
  In5 : Inport  Port=5  LatchInput=off
  Constant : Constant  Value=sg0
  Selector5 : Selector  IndexMode=Zero-based  ElementSrc=External  Elements=[1 3]
  gpe_cell : Subsystem
  synap_gpe : Subsystem
  Out1 : Outport
  Out2 : Outport  Port=2
  wires:
  gpe_cell/1(Out1) -> synap_gpe/1(In1), Out2/1
  In3/1 -> gpe_cell/3(In3)
  In4/1 -> gpe_cell/4(In4)
  synap_gpe/1(Out1) -> Out1/1
  In1/1 -> gpe_cell/1(In1)
  In2/1 -> gpe_cell/2(In2)
  Selector5/1 -> synap_gpe/2(In2)
  In5/1 -> gpe_cell/5(In5), Selector5/2
  Constant/1 -> Selector5/1

== system GPESTN1_GPEDBS/GPE_cell2 ==
  In1 : Inport  Port=1  LatchInput=off
  In2 : Inport  Port=2  LatchInput=off
  In3 : Inport  Port=3  LatchInput=off
  In4 : Inport  Port=4  LatchInput=off
  In5 : Inport  Port=5  LatchInput=off
  Constant : Constant  Value=sg0
  Selector5 : Selector  IndexMode=Zero-based  ElementSrc=External  Elements=[1 3]
  gpe_cell : Subsystem
  synap_gpe : Subsystem
  Out1 : Outport
  Out2 : Outport  Port=2
  wires:
  gpe_cell/1(Out1) -> synap_gpe/1(In1), Out2/1
  In3/1 -> gpe_cell/3(In3)
  In4/1 -> gpe_cell/4(In4)
  synap_gpe/1(Out1) -> Out1/1
  In1/1 -> gpe_cell/1(In1)
  In2/1 -> gpe_cell/2(In2)
  Selector5/1 -> synap_gpe/2(In2)
  In5/1 -> gpe_cell/5(In5), Selector5/2
  Constant/1 -> Selector5/1

== system GPESTN1_GPEDBS/GPE_cell3 ==
  In1 : Inport  Port=1  LatchInput=off
  In2 : Inport  Port=2  LatchInput=off
  In3 : Inport  Port=3  LatchInput=off
  In4 : Inport  Port=4  LatchInput=off
  In5 : Inport  Port=5  LatchInput=off
  Constant : Constant  Value=sg0
  Selector5 : Selector  IndexMode=Zero-based  ElementSrc=External  Elements=[1 3]
  gpe_cell : Subsystem
  synap_gpe : Subsystem
  Out1 : Outport
  Out2 : Outport  Port=2
  wires:
  gpe_cell/1(Out1) -> synap_gpe/1(In1), Out2/1
  In3/1 -> gpe_cell/3(In3)
  In4/1 -> gpe_cell/4(In4)
  synap_gpe/1(Out1) -> Out1/1
  In1/1 -> gpe_cell/1(In1)
  In2/1 -> gpe_cell/2(In2)
  Selector5/1 -> synap_gpe/2(In2)
  In5/1 -> gpe_cell/5(In5), Selector5/2
  Constant/1 -> Selector5/1

== system GPESTN1_GPEDBS/GPE_cell4 ==
  In1 : Inport  Port=1  LatchInput=off
  In2 : Inport  Port=2  LatchInput=off
  In3 : Inport  Port=3  LatchInput=off
  In4 : Inport  Port=4  LatchInput=off
  In5 : Inport  Port=5  LatchInput=off
  Constant : Constant  Value=sg0
  Selector5 : Selector  IndexMode=Zero-based  ElementSrc=External  Elements=[1 3]
  gpe_cell : Subsystem
  synap_gpe : Subsystem
  Out1 : Outport
  Out2 : Outport  Port=2
  wires:
  gpe_cell/1(Out1) -> synap_gpe/1(In1), Out2/1
  In3/1 -> gpe_cell/3(In3)
  In4/1 -> gpe_cell/4(In4)
  synap_gpe/1(Out1) -> Out1/1
  In1/1 -> gpe_cell/1(In1)
  In2/1 -> gpe_cell/2(In2)
  Selector5/1 -> synap_gpe/2(In2)
  In5/1 -> gpe_cell/5(In5), Selector5/2
  Constant/1 -> Selector5/1

== system GPESTN1_GPEDBS/GPE_cell5 ==
  In1 : Inport  Port=1  LatchInput=off
  In2 : Inport  Port=2  LatchInput=off
  In3 : Inport  Port=3  LatchInput=off
  In4 : Inport  Port=4  LatchInput=off
  In5 : Inport  Port=5  LatchInput=off
  Constant : Constant  Value=sg0
  Selector5 : Selector  IndexMode=Zero-based  ElementSrc=External  Elements=[1 3]
  gpe_cell : Subsystem
  synap_gpe : Subsystem
  Out1 : Outport
  Out2 : Outport  Port=2
  wires:
  gpe_cell/1(Out1) -> synap_gpe/1(In1), Out2/1
  In3/1 -> gpe_cell/3(In3)
  In4/1 -> gpe_cell/4(In4)
  synap_gpe/1(Out1) -> Out1/1
  In1/1 -> gpe_cell/1(In1)
  In2/1 -> gpe_cell/2(In2)
  Selector5/1 -> synap_gpe/2(In2)
  In5/1 -> gpe_cell/5(In5), Selector5/2
  Constant/1 -> Selector5/1

== system GPESTN1_GPEDBS/GPE_cell6 ==
  In1 : Inport  Port=1  LatchInput=off
  In2 : Inport  Port=2  LatchInput=off
  In3 : Inport  Port=3  LatchInput=off
  In4 : Inport  Port=4  LatchInput=off
  In5 : Inport  Port=5  LatchInput=off
  Constant : Constant  Value=sg0
  Selector5 : Selector  IndexMode=Zero-based  ElementSrc=External  Elements=[1 3]
  gpe_cell : Subsystem
  synap_gpe : Subsystem
  Out1 : Outport
  Out2 : Outport  Port=2
  wires:
  gpe_cell/1(Out1) -> synap_gpe/1(In1), Out2/1
  In3/1 -> gpe_cell/3(In3)
  In4/1 -> gpe_cell/4(In4)
  synap_gpe/1(Out1) -> Out1/1
  In1/1 -> gpe_cell/1(In1)
  In2/1 -> gpe_cell/2(In2)
  Selector5/1 -> synap_gpe/2(In2)
  In5/1 -> gpe_cell/5(In5), Selector5/2
  Constant/1 -> Selector5/1

== system GPESTN1_GPEDBS/GPE_cell7 ==
  In1 : Inport  Port=1  LatchInput=off
  In2 : Inport  Port=2  LatchInput=off
  In3 : Inport  Port=3  LatchInput=off
  In4 : Inport  Port=4  LatchInput=off
  In5 : Inport  Port=5  LatchInput=off
  Constant : Constant  Value=sg0
  Selector5 : Selector  IndexMode=Zero-based  ElementSrc=External  Elements=[1 3]
  gpe_cell : Subsystem
  synap_gpe : Subsystem
  Out1 : Outport
  Out2 : Outport  Port=2
  wires:
  gpe_cell/1(Out1) -> synap_gpe/1(In1), Out2/1
  In3/1 -> gpe_cell/3(In3)
  In4/1 -> gpe_cell/4(In4)
  synap_gpe/1(Out1) -> Out1/1
  In1/1 -> gpe_cell/1(In1)
  In2/1 -> gpe_cell/2(In2)
  Selector5/1 -> synap_gpe/2(In2)
  In5/1 -> gpe_cell/5(In5), Selector5/2
  Constant/1 -> Selector5/1

== system GPESTN1_GPEDBS/GPE_cell8 ==
  In1 : Inport  Port=1  LatchInput=off
  In2 : Inport  Port=2  LatchInput=off
  In3 : Inport  Port=3  LatchInput=off
  In4 : Inport  Port=4  LatchInput=off
  In5 : Inport  Port=5  LatchInput=off
  Constant : Constant  Value=sg0
  Selector5 : Selector  IndexMode=Zero-based  ElementSrc=External  Elements=[1 3]
  gpe_cell : Subsystem
  synap_gpe : Subsystem
  Out1 : Outport
  Out2 : Outport  Port=2
  wires:
  gpe_cell/1(Out1) -> synap_gpe/1(In1), Out2/1
  In3/1 -> gpe_cell/3(In3)
  In4/1 -> gpe_cell/4(In4)
  synap_gpe/1(Out1) -> Out1/1
  In1/1 -> gpe_cell/1(In1)
  In2/1 -> gpe_cell/2(In2)
  Selector5/1 -> synap_gpe/2(In2)
  In5/1 -> gpe_cell/5(In5), Selector5/2
  Constant/1 -> Selector5/1

== system GPESTN1_GPEDBS/GPE_cell9 ==
  In1 : Inport  Port=1  LatchInput=off
  In2 : Inport  Port=2  LatchInput=off
  In3 : Inport  Port=3  LatchInput=off
  In4 : Inport  Port=4  LatchInput=off
  In5 : Inport  Port=5  LatchInput=off
  Constant : Constant  Value=sg0
  Selector5 : Selector  IndexMode=Zero-based  ElementSrc=External  Elements=[1 3]
  gpe_cell : Subsystem
  synap_gpe : Subsystem
  Out1 : Outport
  Out2 : Outport  Port=2
  wires:
  gpe_cell/1(Out1) -> synap_gpe/1(In1), Out2/1
  In3/1 -> gpe_cell/3(In3)
  In4/1 -> gpe_cell/4(In4)
  synap_gpe/1(Out1) -> Out1/1
  In1/1 -> gpe_cell/1(In1)
  In2/1 -> gpe_cell/2(In2)
  Selector5/1 -> synap_gpe/2(In2)
  In5/1 -> gpe_cell/5(In5), Selector5/2
  Constant/1 -> Selector5/1

== system GPESTN1_GPEDBS/STN_cell1 ==
  In1 : Inport  Port=1  LatchInput=off
  In2 : Inport  Port=2  LatchInput=off
  In3 : Inport  Port=3  LatchInput=off
  In4 : Inport  Port=4  LatchInput=off
  Constant : Constant  Value=ss0
  Selector : Selector  IndexMode=Zero-based  ElementSrc=External  Elements=[1 3]
  Subsystem : Subsystem
  synap_stn : Subsystem
  Out1 : Outport
  Out2 : Outport  Port=2
  wires:
  Subsystem/1(Out1) -> synap_stn/1(In1), Out2/1
  In2/1 -> Subsystem/2(In2)
  In3/1 -> Subsystem/3(In3)
  synap_stn/1(Out1) -> Out1/1
  In1/1 -> Subsystem/1(In1)
  In4/1 -> Subsystem/4(In4), Selector/2
  Selector/1 -> synap_stn/2(In4)
  Constant/1 -> Selector/1

== system GPESTN1_GPEDBS/STN_cell10 ==
  In1 : Inport  Port=1  LatchInput=off
  In2 : Inport  Port=2  LatchInput=off
  In3 : Inport  Port=3  LatchInput=off
  In4 : Inport  Port=4  LatchInput=off
  Constant : Constant  Value=ss0
  Selector : Selector  IndexMode=Zero-based  ElementSrc=External  Elements=[1 3]
  Subsystem : Subsystem
  synap_stn : Subsystem
  Out1 : Outport
  Out2 : Outport  Port=2
  wires:
  Subsystem/1(Out1) -> synap_stn/1(In1), Out2/1
  In2/1 -> Subsystem/2(In2)
  In3/1 -> Subsystem/3(In3)
  synap_stn/1(Out1) -> Out1/1
  In1/1 -> Subsystem/1(In1)
  In4/1 -> Subsystem/4(In4), Selector/2
  Selector/1 -> synap_stn/2(In4)
  Constant/1 -> Selector/1

== system GPESTN1_GPEDBS/STN_cell11 ==
  In1 : Inport  Port=1  LatchInput=off
  In2 : Inport  Port=2  LatchInput=off
  In3 : Inport  Port=3  LatchInput=off
  In4 : Inport  Port=4  LatchInput=off
  Constant : Constant  Value=ss0
  Selector : Selector  IndexMode=Zero-based  ElementSrc=External  Elements=[1 3]
  Subsystem : Subsystem
  synap_stn : Subsystem
  Out1 : Outport
  Out2 : Outport  Port=2
  wires:
  Subsystem/1(Out1) -> synap_stn/1(In1), Out2/1
  In2/1 -> Subsystem/2(In2)
  In3/1 -> Subsystem/3(In3)
  synap_stn/1(Out1) -> Out1/1
  In1/1 -> Subsystem/1(In1)
  In4/1 -> Subsystem/4(In4), Selector/2
  Selector/1 -> synap_stn/2(In4)
  Constant/1 -> Selector/1

== system GPESTN1_GPEDBS/STN_cell12 ==
  In1 : Inport  Port=1  LatchInput=off
  In2 : Inport  Port=2  LatchInput=off
  In3 : Inport  Port=3  LatchInput=off
  In4 : Inport  Port=4  LatchInput=off
  Constant : Constant  Value=ss0
  Selector : Selector  IndexMode=Zero-based  ElementSrc=External  Elements=[1 3]
  Subsystem : Subsystem
  synap_stn : Subsystem
  Out1 : Outport
  Out2 : Outport  Port=2
  wires:
  Subsystem/1(Out1) -> synap_stn/1(In1), Out2/1
  In2/1 -> Subsystem/2(In2)
  In3/1 -> Subsystem/3(In3)
  synap_stn/1(Out1) -> Out1/1
  In1/1 -> Subsystem/1(In1)
  In4/1 -> Subsystem/4(In4), Selector/2
  Selector/1 -> synap_stn/2(In4)
  Constant/1 -> Selector/1

== system GPESTN1_GPEDBS/STN_cell13 ==
  In1 : Inport  Port=1  LatchInput=off
  In2 : Inport  Port=2  LatchInput=off
  In3 : Inport  Port=3  LatchInput=off
  In4 : Inport  Port=4  LatchInput=off
  Constant : Constant  Value=ss0
  Selector : Selector  IndexMode=Zero-based  ElementSrc=External  Elements=[1 3]
  Subsystem : Subsystem
  synap_stn : Subsystem
  Out1 : Outport
  Out2 : Outport  Port=2
  wires:
  Subsystem/1(Out1) -> synap_stn/1(In1), Out2/1
  In2/1 -> Subsystem/2(In2)
  In3/1 -> Subsystem/3(In3)
  synap_stn/1(Out1) -> Out1/1
  In1/1 -> Subsystem/1(In1)
  In4/1 -> Subsystem/4(In4), Selector/2
  Selector/1 -> synap_stn/2(In4)
  Constant/1 -> Selector/1

== system GPESTN1_GPEDBS/STN_cell14 ==
  In1 : Inport  Port=1  LatchInput=off
  In2 : Inport  Port=2  LatchInput=off
  In3 : Inport  Port=3  LatchInput=off
  In4 : Inport  Port=4  LatchInput=off
  Constant : Constant  Value=ss0
  Selector : Selector  IndexMode=Zero-based  ElementSrc=External  Elements=[1 3]
  Subsystem : Subsystem
  synap_stn : Subsystem
  Out1 : Outport
  Out2 : Outport  Port=2
  wires:
  Subsystem/1(Out1) -> synap_stn/1(In1), Out2/1
  In2/1 -> Subsystem/2(In2)
  In3/1 -> Subsystem/3(In3)
  synap_stn/1(Out1) -> Out1/1
  In1/1 -> Subsystem/1(In1)
  In4/1 -> Subsystem/4(In4), Selector/2
  Selector/1 -> synap_stn/2(In4)
  Constant/1 -> Selector/1

== system GPESTN1_GPEDBS/STN_cell15 ==
  In1 : Inport  Port=1  LatchInput=off
  In2 : Inport  Port=2  LatchInput=off
  In3 : Inport  Port=3  LatchInput=off
  In4 : Inport  Port=4  LatchInput=off
  Constant : Constant  Value=ss0
  Selector : Selector  IndexMode=Zero-based  ElementSrc=External  Elements=[1 3]
  Subsystem : Subsystem
  synap_stn : Subsystem
  Out1 : Outport
  Out2 : Outport  Port=2
  wires:
  Subsystem/1(Out1) -> synap_stn/1(In1), Out2/1
  In2/1 -> Subsystem/2(In2)
  In3/1 -> Subsystem/3(In3)
  synap_stn/1(Out1) -> Out1/1
  In1/1 -> Subsystem/1(In1)
  In4/1 -> Subsystem/4(In4), Selector/2
  Selector/1 -> synap_stn/2(In4)
  Constant/1 -> Selector/1

== system GPESTN1_GPEDBS/STN_cell16 ==
  In1 : Inport  Port=1  LatchInput=off
  In2 : Inport  Port=2  LatchInput=off
  In3 : Inport  Port=3  LatchInput=off
  In4 : Inport  Port=4  LatchInput=off
  Constant : Constant  Value=ss0
  Selector : Selector  IndexMode=Zero-based  ElementSrc=External  Elements=[1 3]
  Subsystem : Subsystem
  synap_stn : Subsystem
  Out1 : Outport
  Out2 : Outport  Port=2
  wires:
  Subsystem/1(Out1) -> synap_stn/1(In1), Out2/1
  In2/1 -> Subsystem/2(In2)
  In3/1 -> Subsystem/3(In3)
  synap_stn/1(Out1) -> Out1/1
  In1/1 -> Subsystem/1(In1)
  In4/1 -> Subsystem/4(In4), Selector/2
  Selector/1 -> synap_stn/2(In4)
  Constant/1 -> Selector/1

== system GPESTN1_GPEDBS/STN_cell17 ==
  In1 : Inport  Port=1  LatchInput=off
  In2 : Inport  Port=2  LatchInput=off
  In3 : Inport  Port=3  LatchInput=off
  In4 : Inport  Port=4  LatchInput=off
  Constant : Constant  Value=ss0
  Selector : Selector  IndexMode=Zero-based  ElementSrc=External  Elements=[1 3]
  Subsystem : Subsystem
  synap_stn : Subsystem
  Out1 : Outport
  Out2 : Outport  Port=2
  wires:
  Subsystem/1(Out1) -> synap_stn/1(In1), Out2/1
  In2/1 -> Subsystem/2(In2)
  In3/1 -> Subsystem/3(In3)
  synap_stn/1(Out1) -> Out1/1
  In1/1 -> Subsystem/1(In1)
  In4/1 -> Subsystem/4(In4), Selector/2
  Selector/1 -> synap_stn/2(In4)
  Constant/1 -> Selector/1

== system GPESTN1_GPEDBS/STN_cell2 ==
  In1 : Inport  Port=1  LatchInput=off
  In2 : Inport  Port=2  LatchInput=off
  In3 : Inport  Port=3  LatchInput=off
  In4 : Inport  Port=4  LatchInput=off
  Constant : Constant  Value=ss0
  Selector : Selector  IndexMode=Zero-based  ElementSrc=External  Elements=[1 3]
  Subsystem : Subsystem
  synap_stn : Subsystem
  Out1 : Outport
  Out2 : Outport  Port=2
  wires:
  Subsystem/1(Out1) -> synap_stn/1(In1), Out2/1
  In2/1 -> Subsystem/2(In2)
  In3/1 -> Subsystem/3(In3)
  synap_stn/1(Out1) -> Out1/1
  In1/1 -> Subsystem/1(In1)
  In4/1 -> Subsystem/4(In4), Selector/2
  Selector/1 -> synap_stn/2(In4)
  Constant/1 -> Selector/1

== system GPESTN1_GPEDBS/STN_cell3 ==
  In1 : Inport  Port=1  LatchInput=off
  In2 : Inport  Port=2  LatchInput=off
  In3 : Inport  Port=3  LatchInput=off
  In4 : Inport  Port=4  LatchInput=off
  Constant : Constant  Value=ss0
  Selector : Selector  IndexMode=Zero-based  ElementSrc=External  Elements=[1 3]
  Subsystem : Subsystem
  synap_stn : Subsystem
  Out1 : Outport
  Out2 : Outport  Port=2
  wires:
  Subsystem/1(Out1) -> synap_stn/1(In1), Out2/1
  In2/1 -> Subsystem/2(In2)
  In3/1 -> Subsystem/3(In3)
  synap_stn/1(Out1) -> Out1/1
  In1/1 -> Subsystem/1(In1)
  In4/1 -> Subsystem/4(In4), Selector/2
  Selector/1 -> synap_stn/2(In4)
  Constant/1 -> Selector/1

== system GPESTN1_GPEDBS/STN_cell5 ==
  In1 : Inport  Port=1  LatchInput=off
  In2 : Inport  Port=2  LatchInput=off
  In3 : Inport  Port=3  LatchInput=off
  In4 : Inport  Port=4  LatchInput=off
  Constant : Constant  Value=ss0
  Selector : Selector  IndexMode=Zero-based  ElementSrc=External  Elements=[1 3]
  Subsystem : Subsystem
  synap_stn : Subsystem
  Out1 : Outport
  Out2 : Outport  Port=2
  wires:
  Subsystem/1(Out1) -> synap_stn/1(In1), Out2/1
  In2/1 -> Subsystem/2(In2)
  In3/1 -> Subsystem/3(In3)
  synap_stn/1(Out1) -> Out1/1
  In1/1 -> Subsystem/1(In1)
  In4/1 -> Subsystem/4(In4), Selector/2
  Selector/1 -> synap_stn/2(In4)
  Constant/1 -> Selector/1

== system GPESTN1_GPEDBS/STN_cell6 ==
  In1 : Inport  Port=1  LatchInput=off
  In2 : Inport  Port=2  LatchInput=off
  In3 : Inport  Port=3  LatchInput=off
  In4 : Inport  Port=4  LatchInput=off
  Constant : Constant  Value=ss0
  Selector : Selector  IndexMode=Zero-based  ElementSrc=External  Elements=[1 3]
  Subsystem : Subsystem
  synap_stn : Subsystem
  Out1 : Outport
  Out2 : Outport  Port=2
  wires:
  Subsystem/1(Out1) -> synap_stn/1(In1), Out2/1
  In2/1 -> Subsystem/2(In2)
  In3/1 -> Subsystem/3(In3)
  synap_stn/1(Out1) -> Out1/1
  In1/1 -> Subsystem/1(In1)
  In4/1 -> Subsystem/4(In4), Selector/2
  Selector/1 -> synap_stn/2(In4)
  Constant/1 -> Selector/1

== system GPESTN1_GPEDBS/STN_cell7 ==
  In1 : Inport  Port=1  LatchInput=off
  In2 : Inport  Port=2  LatchInput=off
  In3 : Inport  Port=3  LatchInput=off
  In4 : Inport  Port=4  LatchInput=off
  Constant : Constant  Value=ss0
  Selector : Selector  IndexMode=Zero-based  ElementSrc=External  Elements=[1 3]
  Subsystem : Subsystem
  synap_stn : Subsystem
  Out1 : Outport
  Out2 : Outport  Port=2
  wires:
  Subsystem/1(Out1) -> synap_stn/1(In1), Out2/1
  In2/1 -> Subsystem/2(In2)
  In3/1 -> Subsystem/3(In3)
  synap_stn/1(Out1) -> Out1/1
  In1/1 -> Subsystem/1(In1)
  In4/1 -> Subsystem/4(In4), Selector/2
  Selector/1 -> synap_stn/2(In4)
  Constant/1 -> Selector/1

== system GPESTN1_GPEDBS/STN_cell8 ==
  In1 : Inport  Port=1  LatchInput=off
  In2 : Inport  Port=2  LatchInput=off
  In3 : Inport  Port=3  LatchInput=off
  In4 : Inport  Port=4  LatchInput=off
  Constant : Constant  Value=ss0
  Selector : Selector  IndexMode=Zero-based  ElementSrc=External  Elements=[1 3]
  Subsystem : Subsystem
  synap_stn : Subsystem
  Out1 : Outport
  Out2 : Outport  Port=2
  wires:
  Subsystem/1(Out1) -> synap_stn/1(In1), Out2/1
  In2/1 -> Subsystem/2(In2)
  In3/1 -> Subsystem/3(In3)
  synap_stn/1(Out1) -> Out1/1
  In1/1 -> Subsystem/1(In1)
  In4/1 -> Subsystem/4(In4), Selector/2
  Selector/1 -> synap_stn/2(In4)
  Constant/1 -> Selector/1

== system GPESTN1_GPEDBS/STN_cell9 ==
  In1 : Inport  Port=1  LatchInput=off
  In2 : Inport  Port=2  LatchInput=off
  In3 : Inport  Port=3  LatchInput=off
  In4 : Inport  Port=4  LatchInput=off
  Constant : Constant  Value=ss0
  Selector : Selector  IndexMode=Zero-based  ElementSrc=External  Elements=[1 3]
  Subsystem : Subsystem
  synap_stn : Subsystem
  Out1 : Outport
  Out2 : Outport  Port=2
  wires:
  Subsystem/1(Out1) -> synap_stn/1(In1), Out2/1
  In2/1 -> Subsystem/2(In2)
  In3/1 -> Subsystem/3(In3)
  synap_stn/1(Out1) -> Out1/1
  In1/1 -> Subsystem/1(In1)
  In4/1 -> Subsystem/4(In4), Selector/2
  Selector/1 -> synap_stn/2(In4)
  Constant/1 -> Selector/1

== system GPESTN1_GPEDBS/igpegpe ==
  In1 : Inport  Port=1  LatchInput=off
  In2 : Inport  Port=2  LatchInput=off
  In3 : Inport  Port=3  LatchInput=off
  Fcn : Fcn  Expr=ggpegpe*(u-egpegpe)
  Product : Product  SaturateOnIntegerOverflow=on  InputSameDT=on
  Sum : Sum  SaturateOnIntegerOverflow=on  InputSameDT=on
  Out1 : Outport
  wires:
  Sum/1 -> Product/1
  Fcn/1 -> Product/2
  In1/1 -> Sum/1
  In2/1 -> Sum/2
  Product/1 -> Out1/1
  In3/1 -> Fcn/1

== system GPESTN1_GPEDBS/igpegpe1 ==
  In1 : Inport  Port=1  LatchInput=off
  In2 : Inport  Port=2  LatchInput=off
  In3 : Inport  Port=3  LatchInput=off
  Fcn : Fcn  Expr=ggpegpe*(u-egpegpe)
  Product : Product  SaturateOnIntegerOverflow=on  InputSameDT=on
  Sum : Sum  SaturateOnIntegerOverflow=on  InputSameDT=on
  Out1 : Outport
  wires:
  Sum/1 -> Product/1
  Fcn/1 -> Product/2
  In1/1 -> Sum/1
  In2/1 -> Sum/2
  Product/1 -> Out1/1
  In3/1 -> Fcn/1

== system GPESTN1_GPEDBS/igpegpe10 ==
  In1 : Inport  Port=1  LatchInput=off
  In2 : Inport  Port=2  LatchInput=off
  In3 : Inport  Port=3  LatchInput=off
  Fcn : Fcn  Expr=ggpegpe*(u-egpegpe)
  Product : Product  SaturateOnIntegerOverflow=on  InputSameDT=on
  Sum : Sum  SaturateOnIntegerOverflow=on  InputSameDT=on
  Out1 : Outport
  wires:
  Sum/1 -> Product/1
  Fcn/1 -> Product/2
  In1/1 -> Sum/1
  In2/1 -> Sum/2
  Product/1 -> Out1/1
  In3/1 -> Fcn/1

== system GPESTN1_GPEDBS/igpegpe11 ==
  In1 : Inport  Port=1  LatchInput=off
  In2 : Inport  Port=2  LatchInput=off
  In3 : Inport  Port=3  LatchInput=off
  Fcn : Fcn  Expr=ggpegpe*(u-egpegpe)
  Product : Product  SaturateOnIntegerOverflow=on  InputSameDT=on
  Sum : Sum  SaturateOnIntegerOverflow=on  InputSameDT=on
  Out1 : Outport
  wires:
  Sum/1 -> Product/1
  Fcn/1 -> Product/2
  In1/1 -> Sum/1
  In2/1 -> Sum/2
  Product/1 -> Out1/1
  In3/1 -> Fcn/1

== system GPESTN1_GPEDBS/igpegpe12 ==
  In1 : Inport  Port=1  LatchInput=off
  In2 : Inport  Port=2  LatchInput=off
  In3 : Inport  Port=3  LatchInput=off
  Fcn : Fcn  Expr=ggpegpe*(u-egpegpe)
  Product : Product  SaturateOnIntegerOverflow=on  InputSameDT=on
  Sum : Sum  SaturateOnIntegerOverflow=on  InputSameDT=on
  Out1 : Outport
  wires:
  Sum/1 -> Product/1
  Fcn/1 -> Product/2
  In1/1 -> Sum/1
  In2/1 -> Sum/2
  Product/1 -> Out1/1
  In3/1 -> Fcn/1

== system GPESTN1_GPEDBS/igpegpe13 ==
  In1 : Inport  Port=1  LatchInput=off
  In2 : Inport  Port=2  LatchInput=off
  In3 : Inport  Port=3  LatchInput=off
  Fcn : Fcn  Expr=ggpegpe*(u-egpegpe)
  Product : Product  SaturateOnIntegerOverflow=on  InputSameDT=on
  Sum : Sum  SaturateOnIntegerOverflow=on  InputSameDT=on
  Out1 : Outport
  wires:
  Sum/1 -> Product/1
  Fcn/1 -> Product/2
  In1/1 -> Sum/1
  In2/1 -> Sum/2
  Product/1 -> Out1/1
  In3/1 -> Fcn/1

== system GPESTN1_GPEDBS/igpegpe14 ==
  In1 : Inport  Port=1  LatchInput=off
  In2 : Inport  Port=2  LatchInput=off
  In3 : Inport  Port=3  LatchInput=off
  Fcn : Fcn  Expr=ggpegpe*(u-egpegpe)
  Product : Product  SaturateOnIntegerOverflow=on  InputSameDT=on
  Sum : Sum  SaturateOnIntegerOverflow=on  InputSameDT=on
  Out1 : Outport
  wires:
  Sum/1 -> Product/1
  Fcn/1 -> Product/2
  In1/1 -> Sum/1
  In2/1 -> Sum/2
  Product/1 -> Out1/1
  In3/1 -> Fcn/1

== system GPESTN1_GPEDBS/igpegpe15 ==
  In1 : Inport  Port=1  LatchInput=off
  In2 : Inport  Port=2  LatchInput=off
  In3 : Inport  Port=3  LatchInput=off
  Fcn : Fcn  Expr=ggpegpe*(u-egpegpe)
  Product : Product  SaturateOnIntegerOverflow=on  InputSameDT=on
  Sum : Sum  SaturateOnIntegerOverflow=on  InputSameDT=on
  Out1 : Outport
  wires:
  Sum/1 -> Product/1
  Fcn/1 -> Product/2
  In1/1 -> Sum/1
  In2/1 -> Sum/2
  Product/1 -> Out1/1
  In3/1 -> Fcn/1

== system GPESTN1_GPEDBS/igpegpe2 ==
  In1 : Inport  Port=1  LatchInput=off
  In2 : Inport  Port=2  LatchInput=off
  In3 : Inport  Port=3  LatchInput=off
  Fcn : Fcn  Expr=ggpegpe*(u-egpegpe)
  Product : Product  SaturateOnIntegerOverflow=on  InputSameDT=on
  Sum : Sum  SaturateOnIntegerOverflow=on  InputSameDT=on
  Out1 : Outport
  wires:
  Sum/1 -> Product/1
  Fcn/1 -> Product/2
  In1/1 -> Sum/1
  In2/1 -> Sum/2
  Product/1 -> Out1/1
  In3/1 -> Fcn/1
